simulink model "PIDAdj"  (R2025a)
settings: Solver=FixedStepAuto  StartTime=0.0  StopTime=10.0  FixedStep=1e-4  RelTol=1e-3
settings Model: DataDictionary=PIDControl.sldd  Creator=tecnicomcbti  LastModifiedBy=tecnicomcbti
settings SolverCC: ConcurrentTasks=on  AutoInsertRateTranBlk=on
settings DebuggingCC: UnderspecifiedInitializationDetection=Classic  MergeDetectMultiDrivingBlocksExec=none
settings ModelReferenceCC: PropagateSignalLabelsOutOfModel=off

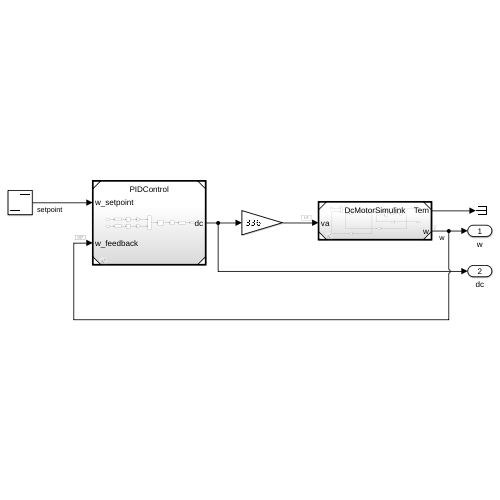
[thumbnail: Simulink's stored preview of the top-level diagram]
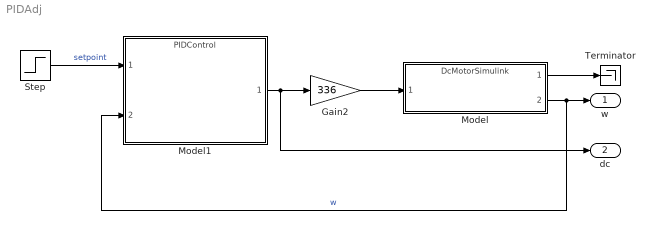
== system PIDAdj ==
  Gain2 : Gain  Gain=336
  Model : ModelReference  ModelNameDialog=DcMotorSimulink.slx  SimulationMode=Normal  ModelReferenceVersion=2.11
  Model1 : ModelReference  ModelNameDialog=PIDControl.slx  SimulationMode=Normal  ModelReferenceVersion=1.6
  Step : Step  Time=0  After=400  SampleTime=1e-3
  Terminator : Terminator
  w : Outport
  dc : Outport  Port=2
  wires:
  Step/1 -> Model1/1  "setpoint"
  Gain2/1 -> Model/1
  Model1/1 -> dc/1, Gain2/1
  Model/2 -> Model1/2, w/1  "w"
  Model/1 -> Terminator/1
